simulink model "different_inverter_controls_BPS"  (R2024b)
settings: Solver=ode4  StartTime=0.0  StopTime=5  FixedStep=Ts  RelTol=1e-3
InitFcn:
  | %mode_of_operation=1;
  | %BESS_control_mode=1;
  | %Gen_Q_Control =1;
  | 
  | %Exciter_init;
  | 
  | %Exciter_init
  | Xq=0.474;
  | %%====================================================
  | % ST6C Exciter Parameters
  | 
  | KPA=30;
  | KIA=59.91;
  | KFF=1;
  | KM=1;
  | KLR=22.47;
  | KCL=1.04;
  | VAMAX=7.05;
  | VAMIN=-6.11;
  | VRMAX=7.05;
  | VRMIN=-6.11;
  | ILR=5.02;
  | KG=1;
  | TG=0.024;
  | TA=0.01;
  | VBMAX=999;
  | VMMAX=7.05;
  | VMMIN=-6.11;
  | KI=0;
  | Kp=1;
  | Kc=0;
  | Vt0=0;
  | VAAMAX=VAMAX;
  | %%========================================================
  | % UEL2C parameters
  | 
  | TUQ=.005;
  | TUP=0.050;
  | TUV=0.2;
  | TQREF=0;
  | Tadj=0;
  | K1=0;
  | K2=2;
  | VBIAS=1;
  | KFB=0;
  | TUL=0;
  | VUImax=1;
  | VUImin=-1;
  | VUELmax1=1;
  | VUELmax2=1;
  | VUELmin1=-1;
  | VUELmin2=-1;
  | KUF=0;
  | KUL=0.24;
  | KUI=0.001;
  | TU1=0;TU2=0;TU3=0;TU4=0;
  | KFIX=1;
  | VF=0;
  | VFB=0;
  | %%===========================================================
  | %OEL3C PARAMETERS
  | ITFpu=1.10;
  | TF=0.02;
  | KSCALE=0.319;
  | K1=1;
  | TOEL=5.00;
  | VOELmax1=0.2353;
  | VOELmax2=0.0;
  | VOELmin1=-0.24;
  | VOELmin2=-1.0;
  | KPOEL=1;
  | KOEL=0.24;
  | %%=============================================================
  | %SCL1C
  | TQSCL=0.012;
  | TIT=0.1;
  | TINV=0;
  | KIUOEX=1;
  | KIUUEX=1;
  | KIOEX=0.0303;
  | KIUEX=0.0303;
  | KPOEX=0;
  | KPUEX=0;
  | VSCLmax=0.20;
  | VSCLmin=-0.10;
  | ISCLIM=1;
  | IQMIN=0.1;
  | K=1;
  | 
  | VAAMAX=VAMAX;
  | Xq=0.474;
  | Ts=5e-5;
  | f=60;
  | Ts_Control = 5e-5;
  | Tbess_Control= 5e-5;
  | 
  | db1=.015;
  | delay=2;
  | KP1=1;
  | KI1=10;
  | KP2=60;
  | KI2=5;
  | KP3=1;
  | KI3=10;
  | KP4=1;
  | KI4=50;
  | KP5=1;
  | KI5=25;
  | Pt_BE_noCC=50e6;
  | Pt_BE_CC=315e6;
  | Qt_BE=35e6;
  | G_ferr=20e6;
  | Qgain_Vref_BESS=20e6;
  | KP6=1;
  | KI6=25;
  | P_t=334e6;
  | clMax=5;
  | clMin=-5;
  | MA_WL=100;
  | TGov=0.02;
values from neighbouring files (symbols this model uses):
  inv1 = struct    [multiInverterParams.m]
  kp_sync = KQ_p/10    (= 0.04)    [multiInverterParams.m]
  Vdc = 1000    [multiInverterParams.m]
  Vpp = 480    [multiInverterParams.m]
undefined symbols (not defined in the file or in its folder): D1, Delta, DiscIntNeverNeededParam, Ion, Lithium, sigbuilder_block, sps
libraries: slpidlib x34, spsThreePhaseVIMeasurementLib x31, spsThreePhaseSeriesRLCBranchLib x23, spsabctodq0Lib x22, spsPower3phInstantaneousLib x22, spsThreePhaseTransformerTwoWindingsLib x16, spsSeriesRLCBranchLib x16, spsThreePhaseSeriesRLCLoadLib x14, simulink x12, spsPLL3phLib x11, spsGroundLib x9, powerlib_extras x8
(part 1 of 9)
settings Model: Creator=mdsha  LastModifiedBy=mdsha
settings DebuggingCC: UnconnectedInputMsg=warning  UnconnectedOutputMsg=warning  UnconnectedLineMsg=warning
settings ModelReferenceCC: EnableRefExpFcnMdlSchedulingChecks=on
settings RTWCC: GPUComputeCapability=3.5  DLArmComputeVersion=19.05

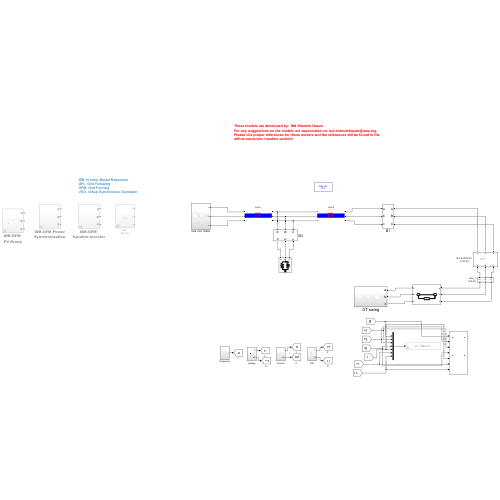
[thumbnail: Simulink's stored preview of the top-level diagram]
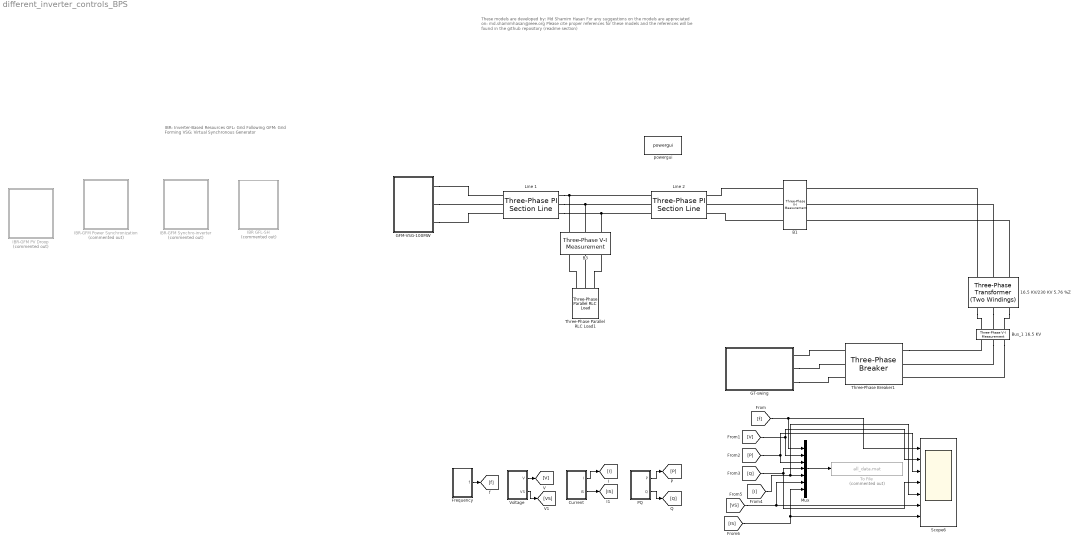
== system different_inverter_controls_BPS ==
  note: IBR: Inverter-Based Resources
      | GFL: Grid Following
      | GFM: Grid Forming
      | VSG: Virtual Synchronous Generator
  note: These models are developed by: Md Shamim Hasan
      | For any suggestions on the models are appreciated on: md.shamimhasan@ieee.org
      | Please cite proper references for these models and the references will be found in the github repository (readme section)
  "16.5 KV/230 KV 5.76 %Z     " : spsThreePhaseTransformerTwoWindingsLib/Three-Phase Transformer (Two Windings)  Winding1Connection=Yg  Winding2Connection=Yg  CoreType=Three single-phase transformers  SetSaturation=off  Hysteresis=off  DataFile='hysteresis'  SetInitialFlux=off  Measurements=None  UNITS=pu  NominalPower=[ 100e6 , f ]  Winding1=[ 16.5e3 , 1e-6, 0 ]  Winding2=[ 345e3 ,1e-6, 0.0576 ]  Rm=500  Lm=500  L0=0.5  Saturation=[ 0,0 ; 0.0024,1.2 ; 1.0,1.52 ]  InitialFluxes=[ 0.8 , -0.8 , 0.7 ]  BreakLoop=off  DiscreteSolver=Trapezoidal iterative  DataType=off  TransfoNumber=1
  B1 : spsThreePhaseVIMeasurementLib/Three-Phase V-I Measurement  VoltageMeasurement=phase-to-ground  SetLabelV=on  LabelV=Vabc_IB  Vpu=on  VpuLL=off  CurrentMeasurement=yes  SetLabelI=on  LabelI=Iabc_IB  Ipu=on  Pbase=100e6  Vbase=345e3  OutputType=Complex  PhasorSimulation=off  PSBequivalent=0
  B3 : spsThreePhaseVIMeasurementLib/Three-Phase V-I Measurement  VoltageMeasurement=phase-to-ground  SetLabelV=on  LabelV=Vabc_load  Vpu=on  VpuLL=off  CurrentMeasurement=yes  SetLabelI=on  LabelI=Iabc_load  Ipu=on  Pbase=100e6  Vbase=345e3  OutputType=Complex  PhasorSimulation=off  PSBequivalent=0
  Bus_1 16.5 KV : spsThreePhaseVIMeasurementLib/Three-Phase V-I Measurement  VoltageMeasurement=phase-to-ground  SetLabelV=on  LabelV=Vabc_1  Vpu=on  VpuLL=off  CurrentMeasurement=yes  SetLabelI=on  LabelI=Iabc_1  Ipu=on  Pbase=50e6  Vbase=16.5e3  OutputType=Complex  PhasorSimulation=off  PSBequivalent=0
  Current : Subsystem
  Frequency : Subsystem
  GFM-VSG-100MW : Subsystem
  GT-swing : Subsystem
  IBR GFL-SH : Subsystem  Commented=on
  IBR-GFM PV Droop : Subsystem  Commented=on
  IBR-GFM Synchro-inverter : Subsystem  Commented=on
  IBR-GFM Power Synchronization : Subsystem  Commented=on
  Line 1 : spsThreePhasePISectionLineLib/Three-Phase PI Section Line  LConnTagsString=a|b|c  RConnTagsString=A|B|C  Length=1  Frequency=f  Resistances=[0.044965 0.11241]  Inductances="[ 1.01e-3  2.02e-3]"  Capacitances=[7.471e-9 4.394e-9]  mask(Three-Phase PI Section Line){}
      mask Display:
      | % This is a new mask on top of the base mask.
      | % Use "View base mask" link below to see the base mask.
      | patch([0.0 0.0 1 1 0.0 0.0 ],[0.4 0.7 0.7 0.4 0.4 0.7],[0 0 1]);
      | patch([0.4 0.4 0.42 0.42],[0.4 0.75 0.75 0.4],[1 0 0]);
      | patch([0.38 0.38 0.57 0.57],[0.7 0.75 0.75 0.7],[1 0 0]);
      | patch([0.53 0.53 0.55 0.55],[0.4 0.75 0.75 0.4],[1 0 0]);
  Line 2 : spsThreePhasePISectionLineLib/Three-Phase PI Section Line  LConnTagsString=a|b|c  RConnTagsString=A|B|C  Length=1  Frequency=f  Resistances=[0.044965 0.11241]  Inductances="[ 1.01e-3  2.02e-3]"  Capacitances=[7.471e-9 4.394e-9]  mask(Three-Phase PI Section Line){}
      mask Display:
      | % This is a new mask on top of the base mask.
      | % Use "View base mask" link below to see the base mask.
      | patch([0.0 0.0 1 1 0.0 0.0 ],[0.4 0.7 0.7 0.4 0.4 0.7],[0 0 1]);
      | patch([0.4 0.4 0.42 0.42],[0.4 0.75 0.75 0.4],[1 0 0]);
      | patch([0.38 0.38 0.57 0.57],[0.7 0.75 0.75 0.7],[1 0 0]);
      | patch([0.53 0.53 0.55 0.55],[0.4 0.75 0.75 0.4],[1 0 0]);
  Mux : Mux  Inputs=7
  PQ : Subsystem
  Scope6 : Scope  NumInputPorts=7
  Three-Phase Parallel RLC Load1 : spsThreePhaseParallelRLCLoadLib/Three-Phase Parallel RLC Load  LConnTagsString=A|B|C  Configuration=Y (grounded)  NominalVoltage=(345000)*1  Vabc=[1e3 1e3 1e3]  Vabcp=[1e3 1e3 1e3]  NominalFrequency=f  UnbalancedPower=off  ActivePower=100e6  InductivePower=44e6  CapacitivePower=0  Pabc=[10e3 9e3 11e3]  QLabc=[100 90 110]  QCabc=[100 90 110]  Pabcp=[10e3 9e3 11e3]  QLabcp=[100 90 110]  QCabcp=[100 90 110]  Measurements=None  LoadType=constant PQ
  Three-Phase Breaker1 : spsThreePhaseBreakerLib/Three-Phase Breaker  InitialState=closed  SwitchA=on  SwitchB=on  SwitchC=on  SwitchTimes=[600 700]  External=off  BreakerResistance=0.01  SnubberResistance=1e6  SnubberCapacitance=inf  Measurements=None
  To File : ToFile  Commented=on  Filename=all_data.mat  MatrixName=all_data  SaveFormat=Timeseries  SampleTime=Ts
  Voltage : Subsystem
  powergui : spspowerguiLib/powergui  Priority=1  SimulationMode=Discrete  SampleTime=Ts  frequency=60  Iterations=50  frequencyindice=0  Pbase=100e6  ErrMax=1e-4  UnitsV=kV  UnitsW=MW  buscounter=0  FunctionMessages=off  echomessages=off  EnableUseOfTLC=off  CurrentSourceSwitches=off  DisableSnubberDevices=off  DisableRonSwitches=off  DisableVfSwitches=off  DisplayEquations=off  AutomaticDiscreteSolvers=off  SolverType=Tustin/Backward Euler (TBE)  Interpol=off  ExternalGateDelay=off  methode=off  Ts=100  x0status=blocks  SPID=on  SwTol=0  HookPort=off  NonlinearTolerance=1e-4  nMaxIteration=100  ContinueOnMaxIteration=off  RestoreLinks=warning  ResistiveCurrentMeasurement=off  Frange=[0:2:500]  Ylog=off  Xlog=on  ShowGrid=off  save=off  variable=ZData  structure=0  ZoomFFT=off  StartTime=0.0  cycles=1  DisplayStyle=1  fundamental=60  FreqAxis=off  MaxFrequency=1000  frequencyindicesteady=1  RmsSteady=1  display=off
  wires:
  Frequency/1(f) -> [f]
  Voltage/1(V) -> [V]
  Current/1(I) -> [I]
  PQ/1(P) -> [P]
  PQ/2(Q) -> [Q]
  [f] -> Scope6/1, Mux/1
  [V] -> Mux/2, Scope6/2
  [P] -> Scope6/3, Mux/3
  [Q] -> Mux/4, Scope6/4
  Mux/1 -> To File/1
  [I] -> Scope6/5, Mux/5
  Current/2(IS) -> [IS]
  Voltage/2(VS) -> [VS]
  [VS] -> Mux/6, Scope6/6
  [IS] -> Scope6/7, Mux/7
  connections:
  Three-Phase Parallel RLC Load1/LConn1 -- B3/RConn1
  Three-Phase Parallel RLC Load1/LConn2 -- B3/RConn2
  Three-Phase Parallel RLC Load1/LConn3 -- B3/RConn3
  Line 1/RConn2 -- Line 2/LConn2 -- B3/LConn2
  Line 1/RConn1 -- Line 2/LConn1 -- B3/LConn1
  Line 1/RConn3 -- Line 2/LConn3 -- B3/LConn3
  B1/RConn1 -- Line 2/RConn1
  B1/RConn2 -- Line 2/RConn2
  B1/RConn3 -- Line 2/RConn3
  Three-Phase Breaker1/RConn1 -- Bus_1 16.5 KV/RConn1
  Three-Phase Breaker1/LConn1 -- GT-swing/RConn1
  GT-swing/RConn2 -- Three-Phase Breaker1/LConn2
  GT-swing/RConn3 -- Three-Phase Breaker1/LConn3
  Bus_1 16.5 KV/RConn3 -- Three-Phase Breaker1/RConn3
  Bus_1 16.5 KV/RConn2 -- Three-Phase Breaker1/RConn2
  "16.5 KV/230 KV 5.76 %Z     "/LConn2 -- Bus_1 16.5 KV/LConn2
  "16.5 KV/230 KV 5.76 %Z     "/LConn3 -- Bus_1 16.5 KV/LConn3
  "16.5 KV/230 KV 5.76 %Z     "/LConn1 -- Bus_1 16.5 KV/LConn1
  "16.5 KV/230 KV 5.76 %Z     "/RConn2 -- B1/LConn2
  "16.5 KV/230 KV 5.76 %Z     "/RConn1 -- B1/LConn1
  "16.5 KV/230 KV 5.76 %Z     "/RConn3 -- B1/LConn3
  GFM-VSG-100MW/RConn1 -- Line 1/LConn1
  GFM-VSG-100MW/RConn2 -- Line 1/LConn2
  GFM-VSG-100MW/RConn3 -- Line 1/LConn3

== system different_inverter_controls_BPS/Current ==
  Gain : Gain  Gain=sqrt(2)
  Mux : Mux  Inputs=3
  RMS : spsRMSLib/RMS  TrueRMS=on  Freq=f  RMSInit=1  Ts=Ts
  Scope : Scope
  Scope1 : Scope
  I : Outport
  IS : Outport  Port=2
  wires:
  RMS/1 -> Gain/1
  Mux/1 -> Scope1/1, IS/1, RMS/1
  Gain/1 -> I/1, Scope/1
  [Iabc_IB] -> Mux/1
  [Iabc_load] -> Mux/2
  [Iabc_BESS_SB] -> Mux/3

== system different_inverter_controls_BPS/Frequency ==
  Mux : Mux  Inputs=3
  PLL (3ph) : spsPLL3phLib/PLL (3ph)  Fmin=45  Par_Init=[0, f]  ParK=[180, 3200, 1]  TcD=1e-4  MaxRateChangeFreq=12  FilterCutOffFreq=25  Ts=Ts  AGC=on
  PLL (3ph)1 : spsPLL3phLib/PLL (3ph)  Fmin=45  Par_Init=[0, f]  ParK=[180, 3200, 1]  TcD=1e-4  MaxRateChangeFreq=12  FilterCutOffFreq=25  Ts=Ts  AGC=on
  PLL (3ph)2 : spsPLL3phLib/PLL (3ph)  Fmin=45  Par_Init=[0, f]  ParK=[180, 3200, 1]  TcD=1e-4  MaxRateChangeFreq=12  FilterCutOffFreq=25  Ts=Ts  AGC=on
  Scope : Scope
  Terminator1 : Terminator
  Terminator2 : Terminator
  Terminator3 : Terminator
  f : Outport
  tag scope: f_system=global
  wires:
  [Vabc_load] -> PLL (3ph)/1
  PLL (3ph)1/2 -> Terminator1/1
  [Vabc_BESS_SB] -> PLL (3ph)1/1
  PLL (3ph)/2 -> Terminator2/1
  [Vabc_IB] -> PLL (3ph)2/1
  PLL (3ph)2/2 -> Terminator3/1
  Mux/1 -> f/1, Scope/1
  PLL (3ph)2/1 -> Mux/1
  PLL (3ph)/1 -> Mux/2
  PLL (3ph)1/1 -> Mux/3, [f_system]

== system different_inverter_controls_BPS/GFM-VSG-100MW ==
  FRT : Subsystem
  IBR-GFM VSG : Subsystem
  a : PMIOPort  Side=Right
  b : PMIOPort  Port=2  Side=Right
  c : PMIOPort  Port=3  Side=Right
  connections:
  IBR-GFM VSG/RConn2 -- FRT/LConn2
  IBR-GFM VSG/RConn1 -- FRT/LConn1
  FRT/RConn1 -- a/RConn1
  FRT/RConn3 -- c/RConn1
  IBR-GFM VSG/RConn3 -- FRT/LConn3
  FRT/RConn2 -- b/RConn1

== system different_inverter_controls_BPS/GT-swing ==
  Gen-a : Subsystem
  Three-Phase V-I Measurement3 : spsThreePhaseVIMeasurementLib/Three-Phase V-I Measurement  VoltageMeasurement=phase-to-ground  SetLabelV=on  LabelV=Vabc_g1  Vpu=on  VpuLL=off  CurrentMeasurement=yes  SetLabelI=on  LabelI=Iabc_g1  Ipu=on  Pbase=100e6  Vbase=16.5e3  OutputType=Complex  PhasorSimulation=off  PSBequivalent=0
  Three-Phase Breaker1 : spsThreePhaseBreakerLib/Three-Phase Breaker  InitialState=closed  SwitchA=on  SwitchB=on  SwitchC=on  SwitchTimes=[600 700]  External=off  BreakerResistance=0.01  SnubberResistance=1e6  SnubberCapacitance=inf  Measurements=None
  a : PMIOPort  Side=Right
  b : PMIOPort  Port=2  Side=Right
  c : PMIOPort  Port=3  Side=Right
  connections:
  Three-Phase V-I Measurement3/RConn1 -- a/RConn1
  Three-Phase V-I Measurement3/RConn2 -- b/RConn1
  Three-Phase V-I Measurement3/RConn3 -- c/RConn1
  Three-Phase Breaker1/RConn1 -- Three-Phase V-I Measurement3/LConn1
  Three-Phase Breaker1/RConn2 -- Three-Phase V-I Measurement3/LConn2
  Three-Phase Breaker1/RConn3 -- Three-Phase V-I Measurement3/LConn3
  Gen-a/RConn2 -- Three-Phase Breaker1/LConn2
  Gen-a/RConn1 -- Three-Phase Breaker1/LConn1
  Gen-a/RConn3 -- Three-Phase Breaker1/LConn3

== system different_inverter_controls_BPS/IBR GFL-SH ==
  BESS : Subsystem  Commented=on  AncestorBlock=|  mask{Pmod=500, Vnom_dc=1000, Bcap=80000, Vnom_prim=16.5e3, Fnom=f, Ts=Ts, Ts_Control=Ts_Control}
      | microgridLibrary/Grid-Connected Battery
      | (Multi-mode EMT Model)
      mask prompts: Pmod "Scale Battery, Multiplier for 100 kW"; Vnom_dc "Nominal Battery Voltage, V"; Bcap "Battery Capacity, Ah"; Vnom_prim "Nominal Grid Connection L-L Voltage, Vrms"; Fnom "Grid Frequency, Fnom [Hz]"; Ts "Simulation Time Step, Ts [s]"; Ts_Control "Controller Time Step, Ts_Control"
      mask init:
      | Pnom = Pmod*100e3;      % Inverter nominal 3-phase power (VA)
      | Vnom_dc = 480;     % Nominal DC link voltage (V)
      | % Vnom_prim = 25e3;  % Nominal inverter primary line-to-line voltage(Vrms)
      | Vnom_sec= 0.85*Vnom_dc/2/sqrt(2)*sqrt(3); % Nominal inverter secondary line-to-line voltage (Vrms)
      | 
      | TotalLeakage = 0.06;   % Transformer total leakage (pu)
      | Rxf = TotalLeakage/25;
      | Lxf = TotalLeakage;
      | 
      | % Inverter choke RL [Rpu Lpu]
      | Rchoke = 0.15/100;
      | Lchoke = 0.15;
      | Zbase = Vnom_sec^2/Pnom;
      | 
      | % Filter C Parameters
      | Qc = 0.1*Pnom;     % Capacitive reactive power (var)
      | Pc = Qc/50;        % Active power (W)      
      | 
      | Clink = 2 * 3/4 * (Pnom/Fnom*2/Vnom_dc^2); % DC link energy for 3/4 cycle of Pnom
      | 
      | % VDC regulator (VDCreg)
      | Kp_VDCreg = 2;           % Proportional gain
      | Ki_VDCreg = 400;        % Integral gain
      | 
      | Rtot_pu = Rxf + Rchoke; % Feedforward values
      | Ltot_pu = Lxf + Lchoke; % Feedforward values
      | 
      | Kp_Ireg = 0.3;          % Proportional gain
      | Ki_Ireg = 20;           % Integral gain
      mask Display: plot(-80,-50,80,50,[0,9,18,24,29,30,29,24,18,9,0,-9,-18,-24,-29,-30,-29,-24,-18,-9,0],[30,29,24,18,9,0,-9,-18,-24,-29,-30,-29,-24,-18,-9,0,9,18,24,29,30],[-50],[0],[50],[0],[45 35 40 40 40],[15 15 15 20 10],[1 2 3 4 5 6 7 8 9 10 11 12 13 14 15 16 17 18 19 20 21].*1.5-15,[0,9,18,24,29,30,29,24,18,9,0,-9,-18,-24,-29,-30,-29,-24,-18,-9,0]./2.4)
  BG1 : spsThreePhaseVIMeasurementLib/Three-Phase V-I Measurement  VoltageMeasurement=phase-to-ground  SetLabelV=on  LabelV=Vabc_BESS_SB  Vpu=on  VpuLL=off  CurrentMeasurement=yes  SetLabelI=on  LabelI=Iabc_BESS_SB  Ipu=on  Pbase=100e6  Vbase=230e3  OutputType=Complex  PhasorSimulation=off  PSBequivalent=0
  BG3 : spsThreePhaseVIMeasurementLib/Three-Phase V-I Measurement  VoltageMeasurement=phase-to-ground  SetLabelV=off  LabelV=Vabc_BESS_SBa  Vpu=on  VpuLL=off  CurrentMeasurement=yes  SetLabelI=off  LabelI=Iabc_BESS_SBa  Ipu=on  Pbase=50e6  Vbase=230e3  OutputType=Complex  PhasorSimulation=off  PSBequivalent=0
  Brk3 : spsThreePhaseBreakerLib/Three-Phase Breaker  InitialState=closed  SwitchA=on  SwitchB=on  SwitchC=on  SwitchTimes=[5 100]*100  External=off  BreakerResistance=0.001  SnubberResistance=inf  SnubberCapacitance=0  Measurements=None
      settings: AttributesFormatString=\n
  Gain : Gain  Gain=sqrt(2)
  IBR : Subsystem  AncestorBlock=|  mask{Pmod=1000, Vnom_dc=1000, Bcap=800000, Vnom_prim=16.5e3, Fnom=f, Ts=Ts, Ts_Control=Ts_Control}
      | microgridLibrary/Grid-Connected Battery
      | (Multi-mode EMT Model)
      mask prompts: Pmod "Scale, Multiplier for 100 kW"; Vnom_dc "Nominal  Voltage, V"; Bcap "Battery Capacity, Ah (If battery is used)"; Vnom_prim "Nominal Grid Connection L-L Voltage, Vrms"; Fnom "Grid Frequency, Fnom [Hz]"; Ts "Simulation Time Step, Ts [s]"; Ts_Control "Controller Time Step, Ts_Control"
      mask init: same as different_inverter_controls_BPS/IBR GFL-SH/BESS
  "Power (3ph, Instantaneous)1" : spsPower3phInstantaneousLib/Power (3ph, Instantaneous)
  RMS : spsRMSLib/RMS  TrueRMS=on  Freq=60  RMSInit=120  Ts=0
  Scope : Scope
  Scope1 : Scope  NumInputPorts=2
  Scope2 : Scope
  Scope3 : Scope
  Terminator : Terminator  Commented=on
  Terminator1 : Terminator
  XFR : spsThreePhaseTransformerTwoWindingsLib/Three-Phase Transformer (Two Windings)  Winding1Connection=Yg  Winding2Connection=Yg  CoreType=Three single-phase transformers  SetSaturation=off  Hysteresis=off  DataFile='hysteresis'  SetInitialFlux=off  Measurements=None  UNITS=pu  NominalPower=[100e6, f ]  Winding1=[16.5e3/sqrt(3), 1e-6, 0.0586 ]  Winding2="[230e3/sqrt(2),  1e-6, 0.0586 ]"  Rm=500  Lm=500  L0=0.5  Saturation=[ 0,0 ; 0.0024,1.2 ; 1.0,1.52 ]  InitialFluxes=[ 0.8 , -0.8 , 0.7 ]  BreakLoop=off  DiscreteSolver=Trapezoidal iterative  DataType=off  TransfoNumber=1
  km Area 2 : spsThreePhasePISectionLineLib/Three-Phase PI Section Line  LConnTagsString=a|b|c  RConnTagsString=A|B|C  Length=1  Frequency=f  Resistances=[0.0001*529 1.61]  Inductances=[0.001*529/(377) 0.0061]  Capacitances=[0.00175/529/(377) 5.2489e-9]
  a : PMIOPort  Side=Right
  b : PMIOPort  Port=2  Side=Right
  c : PMIOPort  Port=3  Side=Right
  wires:
  Gain/1 -> Scope3/1
  RMS/1 -> Gain/1
  [Vabc_BESS_SB] -> Scope/1
  BG3/1 -> Scope2/1, "Power (3ph, Instantaneous)1"/1
  BG3/2 -> "Power (3ph, Instantaneous)1"/2, RMS/1
  "Power (3ph, Instantaneous)1"/1 -> Scope1/1
  "Power (3ph, Instantaneous)1"/2 -> Scope1/2
  BESS/1(m) -> Terminator/1
  IBR/1(m) -> Terminator1/1
  connections:
  km Area 2/RConn1 -- BG3/RConn1
  km Area 2/RConn2 -- BG3/RConn2
  km Area 2/RConn3 -- BG3/RConn3
  km Area 2/LConn3 -- Brk3/RConn3
  km Area 2/LConn1 -- Brk3/RConn1
  km Area 2/LConn2 -- Brk3/RConn2
  BG1/LConn3 -- Brk3/LConn3
  Brk3/LConn2 -- BG1/LConn2
  Brk3/LConn1 -- BG1/LConn1
  BG1/RConn2 -- b/RConn1
  BG1/RConn1 -- a/RConn1
  BG1/RConn3 -- c/RConn1
  XFR/RConn1 -- BG3/LConn1
  XFR/RConn2 -- BG3/LConn2
  XFR/RConn3 -- BG3/LConn3
  IBR/RConn1 -- XFR/LConn1
  IBR/RConn2 -- XFR/LConn2
  IBR/RConn3 -- XFR/LConn3

== system different_inverter_controls_BPS/IBR-GFM PV Droop ==
  BG : spsThreePhaseVIMeasurementLib/Three-Phase V-I Measurement  VoltageMeasurement=phase-to-ground  SetLabelV=on  LabelV=Vabc_BESS_SB  Vpu=on  VpuLL=off  CurrentMeasurement=yes  SetLabelI=on  LabelI=Iabc_BESS_SB  Ipu=on  Pbase=100e6  Vbase=16.5e3  OutputType=Complex  PhasorSimulation=off  PSBequivalent=0
  Ground : spsGroundLib/Ground  Commented=on  LConnTagsString=a
  IBR : Subsystem  AncestorBlock=|  mask{Pmod=1100, Vnom_dc=1000, Bcap=110000, Vnom_prim=16.5e3, Fnom=f, Ts=Ts, Ts_Control=Ts_Control}
      | microgridLibrary/Grid-Connected Battery
      | (Multi-mode EMT Model)
      mask prompts: Pmod "Scale Battery, Multiplier for 100 kW"; Vnom_dc "Nominal Battery Voltage, V"; Bcap "Battery Capacity, Ah"; Vnom_prim "Nominal Grid Connection L-L Voltage, Vrms"; Fnom "Grid Frequency, Fnom [Hz]"; Ts "Simulation Time Step, Ts [s]"; Ts_Control "Controller Time Step, Ts_Control"
      mask init: same as different_inverter_controls_BPS/IBR GFL-SH/BESS
  RC snubber : spsThreePhaseSeriesRLCLoadLib/Three-Phase Series RLC Load  Commented=on  LConnTagsString=A|B|C  Configuration=Y (grounded)  NominalVoltage=110e3  Vabc=[1e3 1e3 1e3]  Vabcp=[1e3 1e3 1e3]  NominalFrequency=f  UnbalancedPower=off  ActivePower=1e6  InductivePower=0  CapacitivePower=0  Pabc=[10e3 9e3 11e3]  QLabc=[100 90 110]  QCabc=[100 90 110]  Pabcp=[10e3 9e3 11e3]  QLabcp=[100 90 110]  QCabcp=[100 90 110]  Measurements=None  LoadType=constant Z
  T2: 100MVA 16.5 kV/110 kV : spsThreePhaseTransformerTwoWindingsLib/Three-Phase Transformer (Two Windings)  Winding1Connection=Yg  Winding2Connection=Yg  CoreType=Three single-phase transformers  SetSaturation=off  Hysteresis=off  DataFile='hysteresis'  SetInitialFlux=off  Measurements=None  UNITS=pu  NominalPower=[ 200e6 f ]  Winding1=[16.5e3 1e-6 0.0586]  Winding2=[230e3 1e-6 0.0586]  Rm=500  Lm=500  L0=0.5  Saturation="[ 0,0  ;  0.005,1.2  ;  1.0,1.4 ]"  InitialFluxes=[ 0.8 , -0.8 , 0.7 ]  BreakLoop=off  DiscreteSolver=Trapezoidal iterative  DataType=off  TransfoNumber=0
  Terminator : Terminator
  Three-Phase Series RLC Branch : spsThreePhaseSeriesRLCBranchLib/Three-Phase Series RLC Branch  Commented=on  LConnTagsString=A|B|C  RConnTagsString=A|B|C  BranchType=R  Resistance=10e10  Inductance=1e-3  Capacitance=1e-6  Measurements=None
  Three-Phase Breaker1 : spsThreePhaseBreakerLib/Three-Phase Breaker  InitialState=closed  SwitchA=on  SwitchB=on  SwitchC=on  SwitchTimes=[600 700]  External=off  BreakerResistance=0.01  SnubberResistance=1e6  SnubberCapacitance=inf  Measurements=None
  a : PMIOPort  Side=Right
  b : PMIOPort  Port=2  Side=Right
  c : PMIOPort  Port=3  Side=Right
  wires:
  IBR/1(m) -> Terminator/1
  connections:
  T2: 100MVA 16.5 kV/110 kV/LConn1 -- BG/RConn1
  Three-Phase Breaker1/RConn3 -- BG/LConn3
  Three-Phase Breaker1/RConn2 -- BG/LConn2
  Three-Phase Breaker1/RConn1 -- BG/LConn1
  T2: 100MVA 16.5 kV/110 kV/LConn2 -- BG/RConn2
  T2: 100MVA 16.5 kV/110 kV/LConn3 -- BG/RConn3
  T2: 100MVA 16.5 kV/110 kV/RConn1 -- RC snubber/LConn1 -- a/RConn1
  T2: 100MVA 16.5 kV/110 kV/RConn2 -- RC snubber/LConn2 -- b/RConn1
  T2: 100MVA 16.5 kV/110 kV/RConn3 -- RC snubber/LConn3 -- c/RConn1
  Three-Phase Series RLC Branch/RConn1 -- Ground/LConn1 -- Three-Phase Series RLC Branch/RConn3 -- Three-Phase Series RLC Branch/RConn2
  IBR/RConn3 -- Three-Phase Breaker1/LConn3
  IBR/RConn2 -- Three-Phase Breaker1/LConn2
  IBR/RConn1 -- Three-Phase Breaker1/LConn1

== system different_inverter_controls_BPS/IBR-GFM Synchro-inverter ==
  BG : spsThreePhaseVIMeasurementLib/Three-Phase V-I Measurement  VoltageMeasurement=phase-to-ground  SetLabelV=on  LabelV=Vabc_BESS_SB  Vpu=on  VpuLL=off  CurrentMeasurement=yes  SetLabelI=on  LabelI=Iabc_BESS_SB  Ipu=on  Pbase=100e6  Vbase=16.5e3  OutputType=Complex  PhasorSimulation=off  PSBequivalent=0
  Ground : spsGroundLib/Ground  Commented=on  LConnTagsString=a
  Inverter : Subsystem  AncestorBlock=|  mask{Pmod=1100, Vnom_dc=1000, Bcap=110000, Vnom_prim=16.5e3, Fnom=f, Ts=Ts, Ts_Control=Ts_Control}
      | microgridLibrary/Grid-Connected Battery
      | (Multi-mode EMT Model)
      mask prompts: Pmod "Scale Battery, Multiplier for 100 kW"; Vnom_dc "Nominal Battery Voltage, V"; Bcap "Battery Capacity, Ah"; Vnom_prim "Nominal Grid Connection L-L Voltage, Vrms"; Fnom "Grid Frequency, Fnom [Hz]"; Ts "Simulation Time Step, Ts [s]"; Ts_Control "Controller Time Step, Ts_Control"
      mask init: same as different_inverter_controls_BPS/IBR GFL-SH/BESS
  RC snubber : spsThreePhaseSeriesRLCLoadLib/Three-Phase Series RLC Load  Commented=on  LConnTagsString=A|B|C  Configuration=Y (grounded)  NominalVoltage=110e3  Vabc=[1e3 1e3 1e3]  Vabcp=[1e3 1e3 1e3]  NominalFrequency=f  UnbalancedPower=off  ActivePower=1e6  InductivePower=0  CapacitivePower=0  Pabc=[10e3 9e3 11e3]  QLabc=[100 90 110]  QCabc=[100 90 110]  Pabcp=[10e3 9e3 11e3]  QLabcp=[100 90 110]  QCabcp=[100 90 110]  Measurements=None  LoadType=constant Z
  T2: 100MVA 16.5 kV/110 kV : spsThreePhaseTransformerTwoWindingsLib/Three-Phase Transformer (Two Windings)  Winding1Connection=Yg  Winding2Connection=Yg  CoreType=Three single-phase transformers  SetSaturation=off  Hysteresis=off  DataFile='hysteresis'  SetInitialFlux=off  Measurements=None  UNITS=pu  NominalPower=[ 200e6 f ]  Winding1=[16.5e3 1e-6 0.0586]  Winding2=[230e3 1e-6 0.0586]  Rm=500  Lm=500  L0=0.5  Saturation="[ 0,0  ;  0.005,1.2  ;  1.0,1.4 ]"  InitialFluxes=[ 0.8 , -0.8 , 0.7 ]  BreakLoop=off  DiscreteSolver=Trapezoidal iterative  DataType=off  TransfoNumber=0
  Terminator : Terminator
  Three-Phase Series RLC Branch : spsThreePhaseSeriesRLCBranchLib/Three-Phase Series RLC Branch  Commented=on  LConnTagsString=A|B|C  RConnTagsString=A|B|C  BranchType=R  Resistance=10e10  Inductance=1e-3  Capacitance=1e-6  Measurements=None
  Three-Phase Breaker1 : spsThreePhaseBreakerLib/Three-Phase Breaker  InitialState=closed  SwitchA=on  SwitchB=on  SwitchC=on  SwitchTimes=[600 700]  External=off  BreakerResistance=0.01  SnubberResistance=1e6  SnubberCapacitance=inf  Measurements=None
  a : PMIOPort  Side=Right
  b : PMIOPort  Port=2  Side=Right
  c : PMIOPort  Port=3  Side=Right
  wires:
  Inverter/1(m) -> Terminator/1
  connections:
  Inverter/RConn1 -- Three-Phase Breaker1/LConn1
  Inverter/RConn2 -- Three-Phase Breaker1/LConn2
  Inverter/RConn3 -- Three-Phase Breaker1/LConn3
  Three-Phase Series RLC Branch/RConn2 -- Three-Phase Series RLC Branch/RConn3 -- Ground/LConn1 -- Three-Phase Series RLC Branch/RConn1
  c/RConn1 -- RC snubber/LConn3 -- T2: 100MVA 16.5 kV/110 kV/RConn3
  b/RConn1 -- RC snubber/LConn2 -- T2: 100MVA 16.5 kV/110 kV/RConn2
  a/RConn1 -- RC snubber/LConn1 -- T2: 100MVA 16.5 kV/110 kV/RConn1
  T2: 100MVA 16.5 kV/110 kV/LConn3 -- BG/RConn3
  T2: 100MVA 16.5 kV/110 kV/LConn2 -- BG/RConn2
  Three-Phase Breaker1/RConn1 -- BG/LConn1
  Three-Phase Breaker1/RConn2 -- BG/LConn2
  Three-Phase Breaker1/RConn3 -- BG/LConn3
  T2: 100MVA 16.5 kV/110 kV/LConn1 -- BG/RConn1

== system different_inverter_controls_BPS/IBR-GFM Power Synchronization ==
  BG : spsThreePhaseVIMeasurementLib/Three-Phase V-I Measurement  VoltageMeasurement=phase-to-ground  SetLabelV=on  LabelV=Vabc_BESS_SB  Vpu=on  VpuLL=off  CurrentMeasurement=yes  SetLabelI=on  LabelI=Iabc_BESS_SB  Ipu=on  Pbase=100e6  Vbase=16.5e3  OutputType=Complex  PhasorSimulation=off  PSBequivalent=0
  Ground : spsGroundLib/Ground  Commented=on  LConnTagsString=a
  Inverter : Subsystem  AncestorBlock=|  mask{Pmod=1100, Vnom_dc=1000, Bcap=110000, Vnom_prim=16.5e3, Fnom=f, Ts=Ts, Ts_Control=Ts_Control}
      | microgridLibrary/Grid-Connected Battery
      | (Multi-mode EMT Model)
      mask prompts: Pmod "Scale Battery, Multiplier for 100 kW"; Vnom_dc "Nominal Battery Voltage, V"; Bcap "Battery Capacity, Ah"; Vnom_prim "Nominal Grid Connection L-L Voltage, Vrms"; Fnom "Grid Frequency, Fnom [Hz]"; Ts "Simulation Time Step, Ts [s]"; Ts_Control "Controller Time Step, Ts_Control"
      mask init: same as different_inverter_controls_BPS/IBR GFL-SH/BESS
  RC snubber : spsThreePhaseSeriesRLCLoadLib/Three-Phase Series RLC Load  Commented=on  LConnTagsString=A|B|C  Configuration=Y (grounded)  NominalVoltage=110e3  Vabc=[1e3 1e3 1e3]  Vabcp=[1e3 1e3 1e3]  NominalFrequency=f  UnbalancedPower=off  ActivePower=1e6  InductivePower=0  CapacitivePower=0  Pabc=[10e3 9e3 11e3]  QLabc=[100 90 110]  QCabc=[100 90 110]  Pabcp=[10e3 9e3 11e3]  QLabcp=[100 90 110]  QCabcp=[100 90 110]  Measurements=None  LoadType=constant Z
  T2: 100MVA 16.5 kV/110 kV : spsThreePhaseTransformerTwoWindingsLib/Three-Phase Transformer (Two Windings)  Winding1Connection=Yg  Winding2Connection=Yg  CoreType=Three single-phase transformers  SetSaturation=off  Hysteresis=off  DataFile='hysteresis'  SetInitialFlux=off  Measurements=None  UNITS=pu  NominalPower=[ 200e6 f ]  Winding1=[16.5e3 1e-6 0.0586]  Winding2=[230e3 1e-6 0.0586]  Rm=500  Lm=500  L0=0.5  Saturation="[ 0,0  ;  0.005,1.2  ;  1.0,1.4 ]"  InitialFluxes=[ 0.8 , -0.8 , 0.7 ]  BreakLoop=off  DiscreteSolver=Trapezoidal iterative  DataType=off  TransfoNumber=0
  Terminator : Terminator
  Three-Phase Series RLC Branch : spsThreePhaseSeriesRLCBranchLib/Three-Phase Series RLC Branch  Commented=on  LConnTagsString=A|B|C  RConnTagsString=A|B|C  BranchType=R  Resistance=10e10  Inductance=1e-3  Capacitance=1e-6  Measurements=None
  Three-Phase Breaker1 : spsThreePhaseBreakerLib/Three-Phase Breaker  InitialState=closed  SwitchA=on  SwitchB=on  SwitchC=on  SwitchTimes=[600 700]  External=off  BreakerResistance=0.01  SnubberResistance=1e6  SnubberCapacitance=inf  Measurements=None
  a : PMIOPort  Side=Right
  b : PMIOPort  Port=2  Side=Right
  c : PMIOPort  Port=3  Side=Right
  wires:
  Inverter/1(m) -> Terminator/1
  connections:
  Inverter/RConn1 -- Three-Phase Breaker1/LConn1
  Inverter/RConn2 -- Three-Phase Breaker1/LConn2
  Inverter/RConn3 -- Three-Phase Breaker1/LConn3
  Three-Phase Series RLC Branch/RConn2 -- Three-Phase Series RLC Branch/RConn3 -- Ground/LConn1 -- Three-Phase Series RLC Branch/RConn1
  c/RConn1 -- RC snubber/LConn3 -- T2: 100MVA 16.5 kV/110 kV/RConn3
  b/RConn1 -- RC snubber/LConn2 -- T2: 100MVA 16.5 kV/110 kV/RConn2
  a/RConn1 -- RC snubber/LConn1 -- T2: 100MVA 16.5 kV/110 kV/RConn1
  T2: 100MVA 16.5 kV/110 kV/LConn3 -- BG/RConn3
  T2: 100MVA 16.5 kV/110 kV/LConn2 -- BG/RConn2
  Three-Phase Breaker1/RConn1 -- BG/LConn1
  Three-Phase Breaker1/RConn2 -- BG/LConn2
  Three-Phase Breaker1/RConn3 -- BG/LConn3
  T2: 100MVA 16.5 kV/110 kV/LConn1 -- BG/RConn1

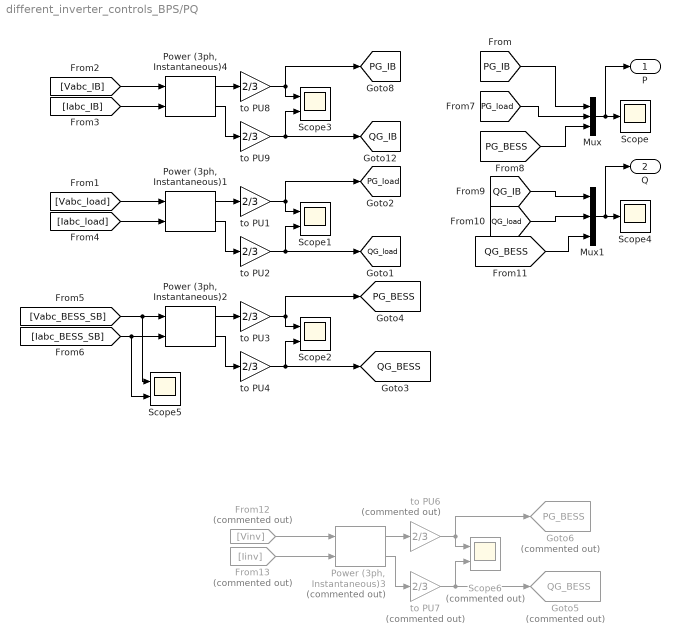
== system different_inverter_controls_BPS/PQ ==
  From12 : From  Commented=on  GotoTag=Vinv  TagVisibility=global
      settings: CloseFcn=tagdialog Close
  From13 : From  Commented=on  GotoTag=Iinv  TagVisibility=global
      settings: CloseFcn=tagdialog Close
  Goto5 : Goto  Commented=on  GotoTag=QG_BESS  TagVisibility=global
  Goto6 : Goto  Commented=on  GotoTag=PG_BESS  TagVisibility=global
  Mux : Mux  Inputs=3
  Mux1 : Mux  Inputs=3
  "Power (3ph, Instantaneous)1" : spsPower3phInstantaneousLib/Power (3ph, Instantaneous)
  "Power (3ph, Instantaneous)2" : spsPower3phInstantaneousLib/Power (3ph, Instantaneous)
  "Power (3ph, Instantaneous)3" : spsPower3phInstantaneousLib/Power (3ph, Instantaneous)  Commented=on
  "Power (3ph, Instantaneous)4" : spsPower3phInstantaneousLib/Power (3ph, Instantaneous)
  Scope : Scope
  Scope{1..3,5} (4 alike) : Scope  NumInputPorts=2
  Scope4 : Scope
  Scope6 : Scope  Commented=on  NumInputPorts=2
  to PU{1..4,8..9} (6 alike) : Gain  Gain=2/3
  to PU6 : Gain  Commented=on  Gain=2/3
  to PU7 : Gain  Commented=on  Gain=2/3
  P : Outport
  Q : Outport  Port=2
  tag scope: PG_BESS=global, PG_IB=global, PG_load=global, QG_BESS=global, QG_IB=global, QG_load=global
  wires:
  to PU9/1 -> Scope3/2, [QG_IB]
  to PU8/1 -> [PG_IB], Scope3/1
  [Iabc_IB] -> "Power (3ph, Instantaneous)4"/2
  "Power (3ph, Instantaneous)4"/2 -> to PU9/1
  "Power (3ph, Instantaneous)4"/1 -> to PU8/1
  [Vabc_IB] -> "Power (3ph, Instantaneous)4"/1
  [Vabc_load] -> "Power (3ph, Instantaneous)1"/1
  "Power (3ph, Instantaneous)1"/1 -> to PU1/1
  "Power (3ph, Instantaneous)1"/2 -> to PU2/1
  [Iabc_load] -> "Power (3ph, Instantaneous)1"/2
  to PU1/1 -> Scope1/1, [PG_load]
  to PU2/1 -> [QG_load], Scope1/2
  to PU4/1 -> Scope2/2, [QG_BESS]
  to PU3/1 -> [PG_BESS], Scope2/1
  [Iabc_BESS_SB] -> Scope5/2, "Power (3ph, Instantaneous)2"/2
  "Power (3ph, Instantaneous)2"/2 -> to PU4/1
  "Power (3ph, Instantaneous)2"/1 -> to PU3/1
  [Vabc_BESS_SB] -> Scope5/1, "Power (3ph, Instantaneous)2"/1
  [PG_IB] -> Mux/1
  [PG_load] -> Mux/2
  [PG_BESS] -> Mux/3
  Mux/1 -> P/1, Scope/1
  Mux1/1 -> Q/1, Scope4/1
  [QG_IB] -> Mux1/1
  [QG_load] -> Mux1/2
  [QG_BESS] -> Mux1/3
  From13/1 -> "Power (3ph, Instantaneous)3"/2
  From12/1 -> "Power (3ph, Instantaneous)3"/1
  "Power (3ph, Instantaneous)3"/1 -> to PU6/1
  to PU6/1 -> Goto6/1, Scope6/1
  to PU7/1 -> Scope6/2, Goto5/1
  "Power (3ph, Instantaneous)3"/2 -> to PU7/1

== system different_inverter_controls_BPS/Voltage ==
  Gain : Gain  Gain=sqrt(2)
  Mux : Mux  Inputs=3
  RMS : spsRMSLib/RMS  TrueRMS=on  Freq=f  RMSInit=1  Ts=Ts
  Scope : Scope
  Scope1 : Scope
  V : Outport
  VS : Outport  Port=2
  wires:
  RMS/1 -> Gain/1
  Mux/1 -> Scope1/1, VS/1, RMS/1
  Gain/1 -> V/1, Scope/1
  [Vabc_BESS_SB] -> Mux/3
  [Vabc_load] -> Mux/2
  [Vabc_IB] -> Mux/1

== system different_inverter_controls_BPS/GFM-VSG-100MW/FRT ==
  B1 : spsThreePhaseVIMeasurementLib/Three-Phase V-I Measurement  VoltageMeasurement=phase-to-ground  SetLabelV=off  LabelV=Vpcc  Vpu=on  VpuLL=off  CurrentMeasurement=yes  SetLabelI=on  LabelI=Iabc_Grid  Ipu=on  Pbase=100e6  Vbase=345e3  OutputType=Complex  PhasorSimulation=off  PSBequivalent=0
  B2 : spsThreePhaseVIMeasurementLib/Three-Phase V-I Measurement  VoltageMeasurement=phase-to-ground  SetLabelV=off  LabelV=V_grid  Vpu=on  VpuLL=off  CurrentMeasurement=yes  SetLabelI=off  LabelI=I_grid  Ipu=on  Pbase=100e6  Vbase=345e3  OutputType=Complex  PhasorSimulation=off  PSBequivalent=0
  Gain1 : Gain  Gain=100e6
  Gain2 : Gain  Gain=100e6
  In -RSY : Subsystem
  Logical Operator : Logic  Operator=NOT  AllPortsSameDT=off  OutDataTypeStr=boolean
  "Power (3ph, Instantaneous)3" : spsPower3phInstantaneousLib/Power (3ph, Instantaneous)
  Scope1 : Scope
  Scope2 : Scope
  Scope3 : Scope
  Scope4 : Scope  NumInputPorts=2
  Three-Phase PI Section Line1 : spsThreePhasePISectionLineLib/Three-Phase PI Section Line  LConnTagsString=a|b|c  RConnTagsString=A|B|C  Length=1  Frequency=f  Resistances=[ 0.01273 0.3864]  Inductances="[ 0.9337e-3  4.1264e-3]"  Capacitances=[12.74e-9 7.751e-9]
  Three-Phase PI Section Line2 : spsThreePhasePISectionLineLib/Three-Phase PI Section Line  LConnTagsString=a|b|c  RConnTagsString=A|B|C  Length=1  Frequency=f  Resistances=[ 0.01273 0.3864]  Inductances="[ 0.9337e-3  4.1264e-3]"  Capacitances=[12.74e-9 7.751e-9]
  Three-Phase Breaker : spsThreePhaseBreakerLib/Three-Phase Breaker  InitialState=closed  SwitchA=on  SwitchB=on  SwitchC=on  SwitchTimes="[5  5.2]*100"  External=on  BreakerResistance=0.01  SnubberResistance=1e6  SnubberCapacitance=inf  Measurements=None
  Three-Phase Fault : spsThreePhaseFaultLib/Three-Phase Fault  InitialStates=0  FaultA=on  FaultB=on  FaultC=on  GroundFault=on  SwitchTimes=[3 3+12/60]  External=off  SwitchStatus=NaN  FaultResistance=0.001  GroundResistance=0.01  SnubberResistance=1e6  SnubberCapacitance=inf  Measurements=None
  a1 : PMIOPort  Side=Left
  b1 : PMIOPort  Port=2  Side=Left
  c1 : PMIOPort  Port=3  Side=Left
  a : PMIOPort  Port=4  Side=Right
  b : PMIOPort  Port=5  Side=Right
  c : PMIOPort  Port=6  Side=Right
  tag scope: P_Slack=global, Q_Slack=global, Vabc_Grid=global, Vabc_PCC=global
  wires:
  "Power (3ph, Instantaneous)3"/1 -> Gain1/1
  "Power (3ph, Instantaneous)3"/2 -> Gain2/1
  Gain2/1 -> [Q_Slack]
  Gain1/1 -> [P_Slack], Scope2/1
  [mode] -> Logical Operator/1, Scope3/1
  [Vabc_PCC] -> In -RSY/2(VPCC)
  B2/2 -> "Power (3ph, Instantaneous)3"/2, [Iabc_PCC]
  [Vabc_Grid] -> In -RSY/1(VGrid)
  Logical Operator/1 -> Three-Phase Breaker/1, Scope1/1
  B1/1 -> [Vabc_Grid]
  B2/1 -> [Vabc_PCC], "Power (3ph, Instantaneous)3"/1
  [Vabc_Grid] -> Scope4/1
  [Vabc_PCC] -> Scope4/2
  connections:
  B2/RConn2 -- Three-Phase Breaker/RConn2
  B2/RConn1 -- Three-Phase Breaker/RConn1
  B2/RConn3 -- Three-Phase Breaker/RConn3
  Three-Phase Breaker/LConn2 -- Three-Phase Fault/LConn2 -- B1/LConn2
  B1/LConn1 -- Three-Phase Fault/LConn1 -- Three-Phase Breaker/LConn1
  Three-Phase Breaker/LConn3 -- Three-Phase Fault/LConn3 -- B1/LConn3
  B2/LConn2 -- Three-Phase PI Section Line2/LConn2
  B2/LConn1 -- Three-Phase PI Section Line2/LConn1
  B2/LConn3 -- Three-Phase PI Section Line2/LConn3
  a1/RConn1 -- Three-Phase PI Section Line2/RConn1
  b1/RConn1 -- Three-Phase PI Section Line2/RConn2
  c1/RConn1 -- Three-Phase PI Section Line2/RConn3
  Three-Phase PI Section Line1/RConn2 -- B1/RConn2
  Three-Phase PI Section Line1/RConn1 -- B1/RConn1
  Three-Phase PI Section Line1/RConn3 -- B1/RConn3
  Three-Phase PI Section Line1/LConn1 -- a/RConn1
  Three-Phase PI Section Line1/LConn2 -- b/RConn1
  Three-Phase PI Section Line1/LConn3 -- c/RConn1

== system different_inverter_controls_BPS/GFM-VSG-100MW/IBR-GFM VSG ==
  BG : spsThreePhaseVIMeasurementLib/Three-Phase V-I Measurement  VoltageMeasurement=phase-to-ground  SetLabelV=on  LabelV=Vabc_BESS_SB  Vpu=on  VpuLL=off  CurrentMeasurement=yes  SetLabelI=on  LabelI=Iabc_BESS_SB  Ipu=on  Pbase=100e6  Vbase=16.5e3  OutputType=Complex  PhasorSimulation=off  PSBequivalent=0
  Ground : spsGroundLib/Ground  Commented=on  LConnTagsString=a
  Inverter : Subsystem  AncestorBlock=|  mask{Pmod=1100, Vnom_dc=1000, Bcap=110000, Vnom_prim=16.5e3, Fnom=f, Ts=Ts, Ts_Control=Ts_Control}
      | microgridLibrary/Grid-Connected Battery
      | (Multi-mode EMT Model)
      mask prompts: Pmod "Scale Battery, Multiplier for 100 kW"; Vnom_dc "Nominal Battery Voltage, V"; Bcap "Battery Capacity, Ah"; Vnom_prim "Nominal Grid Connection L-L Voltage, Vrms"; Fnom "Grid Frequency, Fnom [Hz]"; Ts "Simulation Time Step, Ts [s]"; Ts_Control "Controller Time Step, Ts_Control"
      mask init: same as different_inverter_controls_BPS/IBR GFL-SH/BESS
  RC snubber : spsThreePhaseSeriesRLCLoadLib/Three-Phase Series RLC Load  Commented=on  LConnTagsString=A|B|C  Configuration=Y (grounded)  NominalVoltage=110e3  Vabc=[1e3 1e3 1e3]  Vabcp=[1e3 1e3 1e3]  NominalFrequency=f  UnbalancedPower=off  ActivePower=1e6  InductivePower=0  CapacitivePower=0  Pabc=[10e3 9e3 11e3]  QLabc=[100 90 110]  QCabc=[100 90 110]  Pabcp=[10e3 9e3 11e3]  QLabcp=[100 90 110]  QCabcp=[100 90 110]  Measurements=None  LoadType=constant Z
  T2: 200MVA 16.5 kV/345 kV : spsThreePhaseTransformerTwoWindingsLib/Three-Phase Transformer (Two Windings)  Winding1Connection=Yg  Winding2Connection=Yg  CoreType=Three single-phase transformers  SetSaturation=off  Hysteresis=off  DataFile='hysteresis'  SetInitialFlux=off  Measurements=None  UNITS=pu  NominalPower=[ 200e6 f ]  Winding1=[16.5e3 1e-6 0.0586]  Winding2=[345e3 1e-6 0.0586]  Rm=500  Lm=500  L0=0.5  Saturation="[ 0,0  ;  0.005,1.2  ;  1.0,1.4 ]"  InitialFluxes=[ 0.8 , -0.8 , 0.7 ]  BreakLoop=off  DiscreteSolver=Trapezoidal iterative  DataType=off  TransfoNumber=0
  Terminator : Terminator
  Three-Phase Series RLC Branch : spsThreePhaseSeriesRLCBranchLib/Three-Phase Series RLC Branch  Commented=on  LConnTagsString=A|B|C  RConnTagsString=A|B|C  BranchType=R  Resistance=10e10  Inductance=1e-3  Capacitance=1e-6  Measurements=None
  Three-Phase Breaker1 : spsThreePhaseBreakerLib/Three-Phase Breaker  InitialState=closed  SwitchA=on  SwitchB=on  SwitchC=on  SwitchTimes=[600 700]  External=off  BreakerResistance=0.01  SnubberResistance=1e6  SnubberCapacitance=inf  Measurements=None
  a : PMIOPort  Side=Right
  b : PMIOPort  Port=2  Side=Right
  c : PMIOPort  Port=3  Side=Right
  wires:
  Inverter/1(m) -> Terminator/1
  connections:
  T2: 200MVA 16.5 kV/345 kV/LConn1 -- BG/RConn1
  Three-Phase Breaker1/RConn3 -- BG/LConn3
  Three-Phase Breaker1/RConn2 -- BG/LConn2
  Three-Phase Breaker1/RConn1 -- BG/LConn1
  T2: 200MVA 16.5 kV/345 kV/LConn2 -- BG/RConn2
  T2: 200MVA 16.5 kV/345 kV/LConn3 -- BG/RConn3
  T2: 200MVA 16.5 kV/345 kV/RConn1 -- RC snubber/LConn1 -- a/RConn1
  T2: 200MVA 16.5 kV/345 kV/RConn2 -- RC snubber/LConn2 -- b/RConn1
  T2: 200MVA 16.5 kV/345 kV/RConn3 -- RC snubber/LConn3 -- c/RConn1
  Three-Phase Series RLC Branch/RConn1 -- Ground/LConn1 -- Three-Phase Series RLC Branch/RConn3 -- Three-Phase Series RLC Branch/RConn2
  Inverter/RConn3 -- Three-Phase Breaker1/LConn3
  Inverter/RConn2 -- Three-Phase Breaker1/LConn2
  Inverter/RConn1 -- Three-Phase Breaker1/LConn1

== system different_inverter_controls_BPS/GT-swing/Gen-a ==
  Constant10 : Constant  Value=1.000
  Constant6 : Constant
  Ground : spsGroundLib/Ground  LConnTagsString=a
  Synchronous Machine G2 50 MVA 16.5 kV : Subsystem  AncestorBlock=|  mask(Diesel Generator (Simple)){Pn=350e6, Vn=16.5e3, Fn=f, genType=swing, PQ0=[1.0 1.0], H2=1.7}
      | microgridLibrary/Diesel Generator
      | (GOV, AVR only)
      mask prompts: Pn "Generator Rated Power [W]"; Vn "Rated Voltage [V]"; Fn "Rated Frequency [Hz]"; genType "Load Flow Type"; PQ0 "Initial Power, [P0 Q0] [pu]"; H2 "Inertia Co-efficient [H(s)]"
      mask help:
      | The Diesel Generator block contains a synchronous generator, diesel governor and excitation system to represent the dynamics of a Genset. To inspect the model, look under the block mask (Ctrl + u).
      |
      | The inputs to the basic Diesel generator block are the desired speed reference (in pu) and the desired voltage reference (in pu). The output measurements are contained in a Simulink bus, which can be selected by using the Bus Selector block.
      |
      | Note: The initial generator power must be specified for use for Load Flow analysis.
      mask init:
      | % Extract Initial Active/Reactive Power
      | P0 = PQ0(1);
      | Q0 = PQ0(2);
      | 
      | % Select Load Flow Type
      | genBlock = [gcb '/Synchronous Machine'];
      | currentVals = get_param(genBlock,'MaskValues');
      | currentVals{31} = genType;
      | set_param(genBlock,'MaskValues',currentVals);
      | 
      | % Disable Option if Swing Generator Selected
      | currentEnables = get_param(gcb,'MaskEnables');
      | if strcmp(genType,'swing')
      |     currentEnables{5} = 'off';
      | else
      |     currentEnables{5} = 'on';
      | end
      | set_param(gcb,'MaskEnables',currentEnables);
      mask TypeOptions genType: swing | PQ | PV
      mask Display:
      | %image(imread('diesel.jpg'))
      | color('black')
      | port_label('input',1,'wref (pu)')
      | port_label('input',2,'Vref (pu)')
      | port_label('output',1,'m')
      | port_label('Rconn',1,'A')
      | port_label('Rconn',2,'B')
      | port_label('Rconn',3,'C')
  Three-Phase Series RLC Branch : spsThreePhaseSeriesRLCBranchLib/Three-Phase Series RLC Branch  LConnTagsString=A|B|C  RConnTagsString=A|B|C  BranchType=R  Resistance=1e10  Inductance=0  Capacitance=0  Measurements=Branch currents
  Three-Phase V-I Measurement3 : spsThreePhaseVIMeasurementLib/Three-Phase V-I Measurement  VoltageMeasurement=phase-to-ground  SetLabelV=on  LabelV=Vabc_1a  Vpu=on  VpuLL=off  CurrentMeasurement=yes  SetLabelI=on  LabelI=Iabc_1a  Ipu=on  Pbase=100e6  Vbase=16.5e6  OutputType=Complex  PhasorSimulation=off  PSBequivalent=0
  A : PMIOPort  Side=Right
  B : PMIOPort  Port=2  Side=Right
  C : PMIOPort  Port=3  Side=Right
  wires:
  Constant10/1 -> Synchronous Machine G2 50 MVA 16.5 kV/1(wref (pu))
  Synchronous Machine G2 50 MVA 16.5 kV/1(sms) -> [Gens_measure]
  Constant6/1 -> Synchronous Machine G2 50 MVA 16.5 kV/2(Vref (pu))
  connections:
  Three-Phase Series RLC Branch/LConn1 -- Three-Phase V-I Measurement3/LConn1 -- Synchronous Machine G2 50 MVA 16.5 kV/RConn1
  Three-Phase Series RLC Branch/LConn2 -- Three-Phase V-I Measurement3/LConn2 -- Synchronous Machine G2 50 MVA 16.5 kV/RConn2
  Three-Phase Series RLC Branch/LConn3 -- Three-Phase V-I Measurement3/LConn3 -- Synchronous Machine G2 50 MVA 16.5 kV/RConn3
  Three-Phase Series RLC Branch/RConn1 -- Three-Phase Series RLC Branch/RConn3 -- Ground/LConn1 -- Three-Phase Series RLC Branch/RConn2
  Three-Phase V-I Measurement3/RConn1 -- A/RConn1
  Three-Phase V-I Measurement3/RConn2 -- B/RConn1
  Three-Phase V-I Measurement3/RConn3 -- C/RConn1

== system different_inverter_controls_BPS/IBR GFL-SH/BESS ==
  note: Mode & Batt_Mode was same point in original
  "BESS Reference " : Subsystem
  Battery1 : spsBatteryLib/Battery  BatType=Lithium-Ion  NomV=1000  NomQ=Bcap  SOC=100  Batt_Tr=1  PresetModel=on  MaxQ=80000  MinV=750  FullV=1163.9871  Dis_rate=34782.6087  R=0.000125  Normal_OP=72347.8261  expZone="[1080.3859      3930.4348]"
  Bus Selector : BusSelector  OutputSignals=Vabc,Iabc
  DC Link : Subsystem
  Goto Tag Visibility : GotoTagVisibility  GotoTag=PLL_Freq
  Grid Inverter : Subsystem
  Inverter Control : Subsystem
  Measures : Subsystem
  Power Control Loop : Subsystem  SystemSampleTime=Ts
  Rate Transition2 : RateTransition  OutPortSampleTime=Ts_Control
  Scope : Scope
  A : PMIOPort  Side=Right
  B : PMIOPort  Port=2  Side=Right
  C : PMIOPort  Port=3  Side=Right
  m : Outport  VectorParamsAs1DForOutWhenUnconnected=off
  tag scope: Uref=global
  wires:
  [BESS_PQf_ref] -> Power Control Loop/2(PQref_f)
  Rate Transition2/1 -> Bus Selector/1, Power Control Loop/1(m_PQ)
  Inverter Control/1(Uref) -> [Uref], Scope/1, Grid Inverter/1(Uref)
  Bus Selector/1 -> Inverter Control/1(Vabc_prim)  "<Vabc>"
  Bus Selector/2 -> Inverter Control/2(Iabc_prim)  "<Iabc>"
  Grid Inverter/1(m) -> [m_inv]
  [m_inv] -> Measures/1(Grid)
  [m_batt] -> Measures/2(Battery)
  Measures/1(m) -> m/1
  Battery1/1 -> [m_batt]
  [m_inv] -> Rate Transition2/1
  Power Control Loop/1(Idq_ref) -> Inverter Control/3(Idq_ref)
  connections:
  Battery1/LConn1 -- DC Link/LConn1
  Battery1/LConn2 -- DC Link/LConn2
  Grid Inverter/LConn3 -- DC Link/RConn3
  A/RConn1 -- Grid Inverter/RConn1
  B/RConn1 -- Grid Inverter/RConn2
  C/RConn1 -- Grid Inverter/RConn3
  Grid Inverter/LConn1 -- DC Link/RConn1
  DC Link/RConn2 -- Grid Inverter/LConn2

== system different_inverter_controls_BPS/IBR GFL-SH/IBR ==
  " Reference " : Subsystem
  Bus Selector : BusSelector  OutputSignals=Vabc,Iabc
  DC Link : Subsystem
  DC Voltage Source : spsDCVoltageSourceLib/DC Voltage Source  Amplitude=1000  Measurements=None
  Goto Tag Visibility : GotoTagVisibility  GotoTag=PLL_Freq
  Grid Inverter : Subsystem
  Inverter Control : Subsystem
  Measures : Subsystem
  Power Control Loop : Subsystem  SystemSampleTime=Ts
  Rate Transition2 : RateTransition  OutPortSampleTime=Ts_Control
  Scope : Scope
  A : PMIOPort  Side=Right
  B : PMIOPort  Port=2  Side=Right
  C : PMIOPort  Port=3  Side=Right
  m : Outport  VectorParamsAs1DForOutWhenUnconnected=off
  tag scope: Uref=global
  wires:
  [PQf_ref] -> Power Control Loop/2(PQref_f)
  Rate Transition2/1 -> Bus Selector/1, Power Control Loop/1(m_PQ)
  Inverter Control/1(Uref) -> [Uref], Grid Inverter/1(Uref), Scope/1
  Grid Inverter/1(m) -> [m_inv]
  [m_inv] -> Measures/1(Grid)
  [m_batt] -> Measures/2(IBR)
  Measures/1(m) -> m/1
  [m_inv] -> Rate Transition2/1
  Bus Selector/1 -> Inverter Control/1(Vabc_prim)  "<Vabc>"
  Bus Selector/2 -> Inverter Control/2(Iabc_prim)  "<Iabc>"
  Power Control Loop/1(Idq_ref) -> Inverter Control/3(Idq_ref)
  connections:
  A/RConn1 -- Grid Inverter/RConn1
  B/RConn1 -- Grid Inverter/RConn2
  C/RConn1 -- Grid Inverter/RConn3
  DC Voltage Source/RConn1 -- DC Link/LConn1
  DC Voltage Source/LConn1 -- DC Link/LConn2
  DC Link/RConn1 -- Grid Inverter/LConn1
  DC Link/RConn3 -- Grid Inverter/LConn3
  Grid Inverter/LConn2 -- DC Link/RConn2

== system different_inverter_controls_BPS/IBR-GFM PV Droop/IBR ==
  " Reference " : Subsystem
  "            VDC1" : spsDCVoltageSourceLib/DC Voltage Source  Amplitude=Vdc  Measurements=None
  Battery2 : spsBatteryLib/Battery  Commented=on  BatType=Lithium-Ion  NomV=1000  NomQ=Bcap  SOC=100  Batt_Tr=1  PresetModel=on  MaxQ=110000  MinV=750  FullV=1163.9871  Dis_rate=47826.087  R=9.0909e-05  Normal_OP=99478.2609  expZone="[1080.3859      5404.3478]"
  Bus Selector : BusSelector  OutputSignals=Vabc,Iabc
  DC Link : Subsystem
  From1 : From  Commented=on  GotoTag=m_batt
  From2 : From  Commented=on  GotoTag=m_inv
  Goto Tag Visibility : GotoTagVisibility  GotoTag=PLL_Freq
  Goto3 : Goto  Commented=on  GotoTag=m_batt
  Grid Inverter : Subsystem
  Inverter Control : Subsystem
  Measures : Subsystem  Commented=on
  Power Controller : Subsystem  SystemSampleTime=Ts
  Rate Transition2 : RateTransition  OutPortSampleTime=Ts_Control
  Scope : Scope
  Scope1 : Scope
  Voltage Measurement : spsVoltageMeasurementLib/Voltage Measurement  PhasorSimulation=off  OutputType=Complex  PSBequivalent=0
  A : PMIOPort  Side=Right
  B : PMIOPort  Port=2  Side=Right
  C : PMIOPort  Port=3  Side=Right
  m : Outport  VectorParamsAs1DForOutWhenUnconnected=off
  tag scope: Uref=global
  wires:
  [f_system] -> Power Controller/4(fsys)
  [theta_wt] -> Power Controller/3(Input)
  Power Controller/1(theta) -> Inverter Control/3(theta)
  [m_inv] -> Rate Transition2/1
  Measures/1(m) -> m/1
  From1/1 -> Measures/2(Battery)
  From2/1 -> Measures/1(Grid)
  Grid Inverter/1(m) -> [m_inv]
  Bus Selector/2 -> Inverter Control/2(Iabc_prim)  "<Iabc>"
  Bus Selector/1 -> Inverter Control/1(Vabc_prim)  "<Vabc>"
  Inverter Control/1(Uref) -> Grid Inverter/1(Uref), Scope/1, [Uref]
  Rate Transition2/1 -> Power Controller/1(m_PQ), Bus Selector/1
  [BESS_PQf_ref] -> Power Controller/2(PQref_f)
  Power Controller/2(Vdref) -> Inverter Control/4(Vdref)
  Battery2/1 -> Goto3/1
  Voltage Measurement/1 -> Scope1/1
  [V_inv_mag] -> Power Controller/5(V_inv_mag)
  [V_inv_mag] -> Inverter Control/5(V_inv_mag)
  connections:
  DC Link/RConn2 -- Grid Inverter/LConn2
  Grid Inverter/LConn1 -- Voltage Measurement/LConn1 -- DC Link/RConn1
  C/RConn1 -- Grid Inverter/RConn3
  B/RConn1 -- Grid Inverter/RConn2
  A/RConn1 -- Grid Inverter/RConn1
  Grid Inverter/LConn3 -- Voltage Measurement/LConn2 -- DC Link/RConn3
  DC Link/LConn2 -- "            VDC1"/LConn1
  "            VDC1"/RConn1 -- DC Link/LConn1
